simulink model "SinglePhaseACMotor"  (R2024b)
settings: Solver=FixedStepDiscrete  StartTime=0.0  StopTime=10.0  FixedStep=50e-6  RelTol=1e-3
undefined symbols (not defined in the file): Capacitor, Start
libraries: spsIGBTDiodeLib x4, spsSinglePhaseAsynchronousMachineLib x1, spsDCVoltageSourceLib x1, spsGroundLib x1, sps_lib x1
settings Model: Creator=User  LastModifiedBy=User

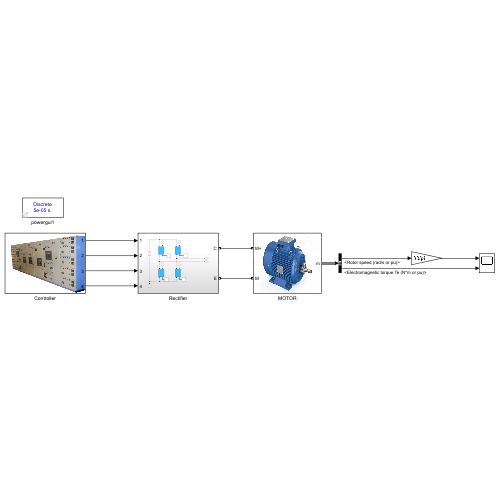
[thumbnail: Simulink's stored preview of the top-level diagram]
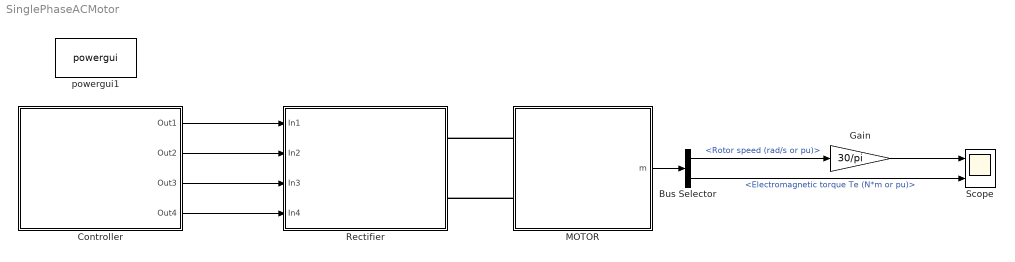
== system SinglePhaseACMotor ==
  Bus Selector : BusSelector  OutputSignals=Mechanical.Rotor speed (rad/s or pu),Mechanical.Electromagnetic torque Te (N*m or pu)
  Controller : Subsystem
      mask Display: image('cpri-approved-electrical-control-panels-1000x1000.jpg');
  Gain : Gain  Gain=30/pi
  MOTOR : Subsystem
      mask Display: image('depositphotos_72535859-stock-photo-blue-industrial-electric-motor.jpg');
  Rectifier : Subsystem
  Scope : Scope  NumInputPorts=2
  powergui1 : sps_lib/powergui  Priority=1  SimulationMode=Discrete  SampleTime=50e-6  frequency=60  Iterations=50  frequencyindice=60  Pbase=100e6  ErrMax=1e-4  UnitsV=kV  UnitsW=MW  buscounter=0  FunctionMessages=off  echomessages=off  EnableUseOfTLC=off  CurrentSourceSwitches=off  DisableSnubberDevices=off  DisableRonSwitches=off  DisableVfSwitches=off  DisplayEquations=off  AutomaticDiscreteSolvers=off  SolverType=Tustin/Backward Euler (TBE)  Interpol=off  ExternalGateDelay=off  methode=off  Ts=100  x0status=blocks  SPID=on  SwTol=0  HookPort=off  NonlinearTolerance=1e-4  nMaxIteration=100  ContinueOnMaxIteration=off  RestoreLinks=warning  ResistiveCurrentMeasurement=off  Frange=[0:2:500]  Ylog=off  Xlog=on  ShowGrid=off  save=off  variable=ZData  structure=0  ZoomFFT=off  StartTime=0.0  cycles=1  DisplayStyle=1  fundamental=60  FreqAxis=off  MaxFrequency=1000  frequencyindicesteady=1  RmsSteady=1  display=off
  wires:
  Bus Selector/1 -> Gain/1  "<Rotor speed (rad/s or pu)>"
  Gain/1 -> Scope/1
  Bus Selector/2 -> Scope/2  "<Electromagnetic torque Te (N*m or pu)>"
  Controller/1(Out1) -> Rectifier/1(In1)
  Controller/2(Out2) -> Rectifier/2(In2)
  Controller/3(Out3) -> Rectifier/3(In3)
  Controller/4(Out4) -> Rectifier/4(In4)
  MOTOR/1(m) -> Bus Selector/1
  connections:
  MOTOR/LConn1 -- Rectifier/RConn1
  MOTOR/LConn2 -- Rectifier/RConn2

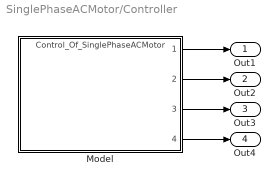
== system SinglePhaseACMotor/Controller ==
  Model : ModelReference  ModelNameDialog=Control_Of_SinglePhaseACMotor.slx  SimulationMode=Normal  ModelReferenceVersion=1.3
  Out1 : Outport
  Out2 : Outport  Port=2
  Out3 : Outport  Port=3
  Out4 : Outport  Port=4
  wires:
  Model/1 -> Out1/1
  Model/2 -> Out2/1
  Model/3 -> Out3/1
  Model/4 -> Out4/1

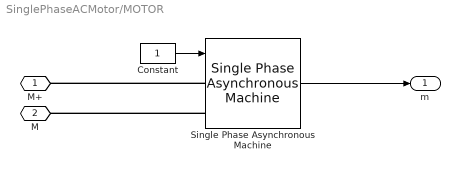
== system SinglePhaseACMotor/MOTOR ==
  Constant : Constant
  Single Phase Asynchronous Machine : spsSinglePhaseAsynchronousMachineLib/Single Phase Asynchronous Machine  MechanicalLoad=Torque Tm  UNITS=SI  MachineType=Capacitor-Start  MeasurementBus=off  NominalParameters="[ .25*746  110  60]"  MainWindingStator="[2.02  7.4e-3]"  MainWindingRotor="[4.12  5.6e-3]"  MutualInductance=0.1772  AuxiliaryWinding="[7.14  8.5e-3]"  Mechanical="[0.0146  0  2 1.18]"  CapacitorStart="[2  254.7e-6]"  CapacitorRun="[18  21.1e-6]"  DisconnectionSpeed=75  InitialSpeed=0  DataType=SI  TsPowergui=0  TsBlock=-1
      settings: LibrarySourceBlock=|
      | sps_lib/Electrical Machines/Single Phase
      | Asynchronous Machine
  M+ : PMIOPort  Side=Left
  M : PMIOPort  Port=2  Side=Left
  m : Outport
  wires:
  Single Phase Asynchronous Machine/1 -> m/1
  Constant/1 -> Single Phase Asynchronous Machine/1
  connections:
  Single Phase Asynchronous Machine/LConn2 -- M/RConn1
  Single Phase Asynchronous Machine/LConn1 -- M+/RConn1

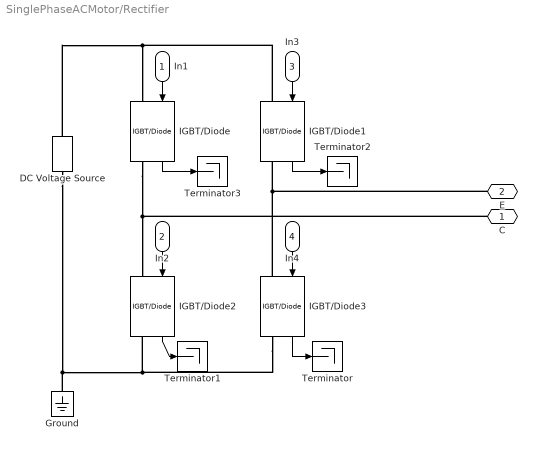
== system SinglePhaseACMotor/Rectifier ==
  In1 : Inport
  In2 : Inport  Port=2
  In3 : Inport  Port=3
  In4 : Inport  Port=4
  DC Voltage Source : spsDCVoltageSourceLib/DC Voltage Source  Amplitude=540  Measurements=None
  Ground : spsGroundLib/Ground  LConnTagsString=a
  IGBT/Diode{,1..3} (4 alike) : spsIGBTDiodeLib/IGBT//Diode  Ron=1e-3  Rs=1e5  Cs=inf  Measurements=on
  Terminator{,1..3} (4 alike) : Terminator
  C : PMIOPort  Side=Right
  E : PMIOPort  Port=2  Side=Right
  wires:
  In3/1 -> IGBT/Diode1/1
  In1/1 -> IGBT/Diode/1
  In2/1 -> IGBT/Diode2/1
  In4/1 -> IGBT/Diode3/1
  IGBT/Diode/1 -> Terminator3/1
  IGBT/Diode1/1 -> Terminator2/1
  IGBT/Diode3/1 -> Terminator/1
  IGBT/Diode2/1 -> Terminator1/1
  connections:
  DC Voltage Source/RConn1 -- IGBT/Diode1/LConn1 -- IGBT/Diode/LConn1
  IGBT/Diode/RConn1 -- C/RConn1 -- IGBT/Diode2/LConn1
  IGBT/Diode3/LConn1 -- E/RConn1 -- IGBT/Diode1/RConn1
  DC Voltage Source/LConn1 -- Ground/LConn1 -- IGBT/Diode2/RConn1 -- IGBT/Diode3/RConn1
